simulink model "PowerFlow_lab_exercise_2024"  (R2024a)
settings: Solver=ode23tb  StartTime=0.0  StopTime=0.5  MaxStep=0.04  RelTol=1e-3  EnableMultiTasking=on
undefined symbols (not defined in the file): D1, Delta
libraries: spsThreePhaseVIMeasurementLib x11, spsLoadFlowBusLib x6, spsThreePhasePISectionLineLib x5, spsRMSLib x5, spsThreePhaseParallelRLCLoadLib x4, spsThreePhaseSourceLib x2, spsThreePhaseTransformerTwoWindingsLib x1, spspowerguiLib x1
Description:
  | Copyright 2008-2019 The MathWorks, Inc.
settings Model: Creator=MathWorks  LastModifiedBy=adysk
settings SolverCC: AlgebraicLoopSolver=TrustRegion
settings DataIOCC: LimitDataPoints=on  SaveFormat=Array  SignalLoggingSaveFormat=ModelDataLogs  ReturnWorkspaceOutputs=off
settings OptimizationCC: ExpressionDepthLimit=2147483647  LifeSpan=inf
settings DebuggingCC: UnderspecifiedInitializationDetection=Classic  MergeDetectMultiDrivingBlocksExec=none  SolverPrmCheckMsg=warning  FcnCallInpInsideContextMsg=warning  StateNameClashWarn=warning  SFUnexpectedBacktrackingDiag=warning  SFNoUnconditionalDefaultTransitionDiag=warning  SFExecutionAtInitializationDiag=none  ArithmeticOperatorsInVariantConditions=warning
settings HardwareCC: ProdBitPerPointer=32  ProdBitPerSizeT=32  ProdBitPerPtrDiffT=32  ProdLargestAtomicFloat=None  ProdIntDivRoundTo=Undefined  ProdEndianess=Unspecified  ProdWordSize=32  ProdHWDeviceType=32-bit Generic
settings ModelReferenceCC: EnableRefExpFcnMdlSchedulingChecks=on  PropagateSignalLabelsOutOfModel=off
settings SFSimCC: SimUseLocalCustomCode=off  CustomCodeUndefinedFunction=UseInterfaceOnly
settings RTWCC: RTWUseLocalCustomCode=off  GPUComputeCapability=3.5  DLArmComputeVersion=19.05
settings CodeAppCC: StateflowObjectComments=on
settings GRTTargetCC: TargetLangStandard=C89/C90 (ANSI)  CombineOutputUpdateFcns=off  GRTInterface=on
settings ConfigComp: CovMetricSettings=dw  CovSaveCumulativeToWorkspaceVar=on  CovSaveSingleToWorkspaceVar=on  CovExternalEMLEnable=off  CovSFcnEnable=off
settings SimscapeCC: SimscapeNormalizeSystem=off

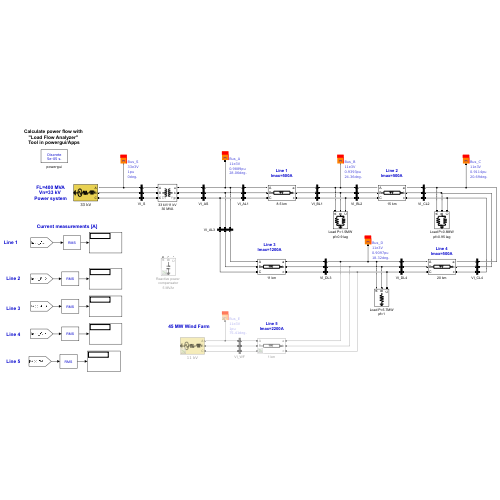
[thumbnail: Simulink's stored preview of the top-level diagram]
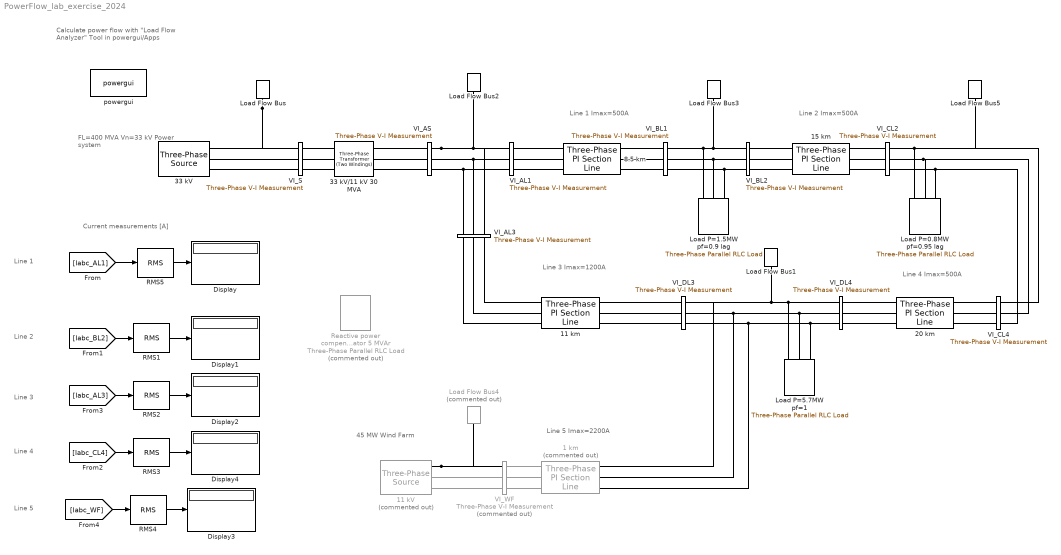
== system PowerFlow_lab_exercise_2024 ==
  note: Line 1
      | Imax=500A
  note: Current measurements [A]
  note: FL=400 MVA
      | Vn=33 kV
      | Power system
  note: Calculate power flow with
      | "Load Flow Analyzer"
      | Tool in powergui/Apps
  note: Line 2
      | Imax=500A
  note: Line 4
      | Imax=500A
  note: Line 3
      | Imax=1200A
  note: Line 1
  note: Line 2
  note: Line 3
  note: Line 4
  note: Line 5
  note: Line 5
      | Imax=2200A
  note: 45 MW Wind Farm
  1 km : spsThreePhasePISectionLineLib/Three-Phase PI Section Line  Commented=on  LConnTagsString=a|b|c  RConnTagsString=A|B|C  Length=1  Frequency=50  Resistances=[0.1153 0.413]  Inductances=[1.05e-3 3.32e-3]  Capacitances=[11.33e-009 5.01e-009]
  11 kV : spsThreePhaseSourceLib/Three-Phase Source  Commented=on  InternalConnection=Yg  VoltagePhases=off  Voltage=(11000)*1.29795  PhaseAngle=102.4466  Voltage_phases=[25e3 25e3 25e3]/sqrt(3)  PhaseAngles_phases=[0 -120 +120]  Frequency=50  NonIdealSource=on  SpecifyImpedance=on  Resistance=0.8929  Inductance=16.58e-3  ShortCircuitLevel=50e6  BaseVoltage=11e3  XRratio=7  BusType=PV  Pref=30000000  Qref=3000000  Prefabc=[10e3, 10e3, 10e3]  Qrefabc=[0, 0, 0]  Qmin=-20000000  Qmax=20000000
  11 km : spsThreePhasePISectionLineLib/Three-Phase PI Section Line  LConnTagsString=a|b|c  RConnTagsString=A|B|C  Length=11  Frequency=50  Resistances=[0.1153 0.413]  Inductances=[1.05e-3 3.32e-3]  Capacitances=[11.33e-009 5.01e-009]
  15 km : spsThreePhasePISectionLineLib/Three-Phase PI Section Line  LConnTagsString=a|b|c  RConnTagsString=A|B|C  Length=15  Frequency=50  Resistances=[0.1153 0.413]  Inductances=[1.05e-3 3.32e-3]  Capacitances=[11.33e-009 5.01e-009]
  20 km : spsThreePhasePISectionLineLib/Three-Phase PI Section Line  LConnTagsString=a|b|c  RConnTagsString=A|B|C  Length=20  Frequency=50  Resistances=[0.1153 0.413]  Inductances=[1.05e-3 3.32e-3]  Capacitances=[11.33e-009 5.01e-009]
  33 kV : spsThreePhaseSourceLib/Three-Phase Source  InternalConnection=Yg  VoltagePhases=off  Voltage=(33000)*1.00988  PhaseAngle=1.1485  Voltage_phases=[25e3 25e3 25e3]/sqrt(3)  PhaseAngles_phases=[0 -120 +120]  Frequency=50  NonIdealSource=on  SpecifyImpedance=on  Resistance=0.8929  Inductance=16.58e-3  ShortCircuitLevel=400e6  BaseVoltage=33e3  XRratio=7  BusType=swing  Pref=10000000  Qref=3000000  Prefabc=[10e3, 10e3, 10e3]  Qrefabc=[0, 0, 0]  Qmin=-Inf  Qmax=Inf
  33 kV/11 kV 30 MVA : spsThreePhaseTransformerTwoWindingsLib/Three-Phase Transformer (Two Windings)  Winding1Connection=Delta (D1)  Winding2Connection=Yg  CoreType=Three single-phase transformers  SetSaturation=off  Hysteresis=off  DataFile='basic_model'  SetInitialFlux=off  Measurements=None  UNITS=pu  NominalPower=[30e6 50 ]  Winding1="[33e3  0.002    0.06 ]"  Winding2="[ 11e3  0.002  0.06]"  Rm=5000  Lm=500  L0=0.5  Saturation="[ 0,0  ;  0.005,1.2  ;  1.0,1.4 ]"  InitialFluxes=[ 0.8 , -0.8 , 0.7 ]  BreakLoop=off  DiscreteSolver=Trapezoidal iterative  DataType=off  TransfoNumber=0
  8.5 km : spsThreePhasePISectionLineLib/Three-Phase PI Section Line  LConnTagsString=a|b|c  RConnTagsString=A|B|C  Length=8.5  Frequency=50  Resistances=[0.1153 0.413]  Inductances=[1.05e-3 3.32e-3]  Capacitances=[11.33e-009 5.01e-009]
  Display{,1..4} (5 alike) : Display
  Load Flow Bus : spsLoadFlowBusLib/Load Flow Bus  LConnTagsString=a  Phases=single  Connectors=on one side  ID=Bus_S  Vbase=33e3  Vref=1  Vangle=0  VLF=1  VLFb=1  VLFc=1  angleLF=0  angleLFb=0  angleLFc=0
      settings: AttributesFormatString=%<ID>\n%<Vbase>V\n%<VLF>pu\n%<angleLF>deg.
  Load Flow Bus1 : spsLoadFlowBusLib/Load Flow Bus  LConnTagsString=a  Phases=single  Connectors=on one side  ID=Bus_D  Vbase=11e3  Vref=1  Vangle=0  VLF=0.9097  VLFb=1  VLFc=1  angleLF=18.32  angleLFb=0  angleLFc=0
      settings: AttributesFormatString=%<ID>\n%<Vbase>V\n%<VLF>pu\n%<angleLF>deg.
  Load Flow Bus2 : spsLoadFlowBusLib/Load Flow Bus  LConnTagsString=a  Phases=single  Connectors=on one side  ID=Bus_A  Vbase=11e3  Vref=1  Vangle=0  VLF=0.9889  VLFb=1  VLFc=1  angleLF=28.06  angleLFb=0  angleLFc=0
      settings: AttributesFormatString=%<ID>\n%<Vbase>V\n%<VLF>pu\n%<angleLF>deg.
  Load Flow Bus3 : spsLoadFlowBusLib/Load Flow Bus  LConnTagsString=a  Phases=single  Connectors=on one side  ID=Bus_B  Vbase=11e3  Vref=1  Vangle=0  VLF=0.9393  VLFb=1  VLFc=1  angleLF=24.36  angleLFb=0  angleLFc=0
      settings: AttributesFormatString=%<ID>\n%<Vbase>V\n%<VLF>pu\n%<angleLF>deg.
  Load Flow Bus4 : spsLoadFlowBusLib/Load Flow Bus  Commented=on  LConnTagsString=a  Phases=single  Connectors=on one side  ID=Bus_E  Vbase=11e3  Vref=1.  Vangle=0  VLF=1  VLFb=1  VLFc=1  angleLF=75.41  angleLFb=0  angleLFc=0
      settings: AttributesFormatString=%<ID>\n%<Vbase>V\n%<VLF>pu\n%<angleLF>deg.
  Load Flow Bus5 : spsLoadFlowBusLib/Load Flow Bus  LConnTagsString=a  Phases=single  Connectors=on one side  ID=Bus_C  Vbase=11e3  Vref=1  Vangle=0  VLF=0.9114  VLFb=1  VLFc=1  angleLF=20.69  angleLFb=0  angleLFc=0
      settings: AttributesFormatString=%<ID>\n%<Vbase>V\n%<VLF>pu\n%<angleLF>deg.
  Load P=0.8MW pf=0.95 lag : spsThreePhaseParallelRLCLoadLib/Three-Phase Parallel RLC Load  LConnTagsString=A|B|C  Configuration=Y (grounded)  NominalVoltage=(11000)*0.911414  Vabc=[1e3 1e3 1e3]  Vabcp=[1e3 1e3 1e3]  NominalFrequency=50  UnbalancedPower=off  ActivePower=800000  InductivePower=262950  CapacitivePower=0  Pabc=[10e3 9e3 11e3]  QLabc=[100 90 110]  QCabc=[100 90 110]  Pabcp=[10e3 9e3 11e3]  QLabcp=[100 90 110]  QCabcp=[100 90 110]  Measurements=None  LoadType=constant PQ
  Load P=1.5MW pf=0.9 lag : spsThreePhaseParallelRLCLoadLib/Three-Phase Parallel RLC Load  LConnTagsString=A|B|C  Configuration=Y (grounded)  NominalVoltage=(11000)*0.939268  Vabc=[1e3 1e3 1e3]  Vabcp=[1e3 1e3 1e3]  NominalFrequency=50  UnbalancedPower=off  ActivePower=1500000  InductivePower=726500  CapacitivePower=0  Pabc=[10e3 9e3 11e3]  QLabc=[100 90 110]  QCabc=[100 90 110]  Pabcp=[10e3 9e3 11e3]  QLabcp=[100 90 110]  QCabcp=[100 90 110]  Measurements=None  LoadType=constant PQ
  Load P=5.7MW pf=1 : spsThreePhaseParallelRLCLoadLib/Three-Phase Parallel RLC Load  LConnTagsString=A|B|C  Configuration=Y (grounded)  NominalVoltage=(11000)*0.9097  Vabc=[1e3 1e3 1e3]  Vabcp=[1e3 1e3 1e3]  NominalFrequency=50  UnbalancedPower=off  ActivePower=5700000  InductivePower=0  CapacitivePower=0  Pabc=[10e3 9e3 11e3]  QLabc=[100 90 110]  QCabc=[100 90 110]  Pabcp=[10e3 9e3 11e3]  QLabcp=[100 90 110]  QCabcp=[100 90 110]  Measurements=None  LoadType=constant PQ
  RMS{1..5} (5 alike) : spsRMSLib/RMS  TrueRMS=on  Freq=50  RMSInit=120  Ts=0
  Reactive power compensator 5 MVAr : spsThreePhaseParallelRLCLoadLib/Three-Phase Parallel RLC Load  Commented=on  LConnTagsString=A|B|C  Configuration=Y (grounded)  NominalVoltage=(11000)*0.943215  Vabc=[1e3 1e3 1e3]  Vabcp=[1e3 1e3 1e3]  NominalFrequency=50  UnbalancedPower=off  ActivePower=0  InductivePower=0  CapacitivePower=5000000  Pabc=[10e3 9e3 11e3]  QLabc=[100 90 110]  QCabc=[100 90 110]  Pabcp=[10e3 9e3 11e3]  QLabcp=[100 90 110]  QCabcp=[100 90 110]  Measurements=None  LoadType=constant PQ
  VI_AL1 : spsThreePhaseVIMeasurementLib/Three-Phase V-I Measurement  VoltageMeasurement=phase-to-ground  SetLabelV=on  LabelV=Vabc_AL1  Vpu=off  VpuLL=off  CurrentMeasurement=yes  SetLabelI=on  LabelI=Iabc_AL1  Ipu=off  Pbase=10e6  Vbase=25e3  OutputType=Complex  PhasorSimulation=off  PSBequivalent=0
  VI_AL3 : spsThreePhaseVIMeasurementLib/Three-Phase V-I Measurement  VoltageMeasurement=phase-to-ground  SetLabelV=on  LabelV=Vabc_AL3  Vpu=off  VpuLL=off  CurrentMeasurement=yes  SetLabelI=on  LabelI=Iabc_AL3  Ipu=off  Pbase=10e6  Vbase=25e3  OutputType=Complex  PhasorSimulation=off  PSBequivalent=0
  VI_AS : spsThreePhaseVIMeasurementLib/Three-Phase V-I Measurement  VoltageMeasurement=phase-to-ground  SetLabelV=on  LabelV=Vabc_AS  Vpu=off  VpuLL=off  CurrentMeasurement=yes  SetLabelI=on  LabelI=Iabc_AS  Ipu=off  Pbase=10e6  Vbase=25e3  OutputType=Complex  PhasorSimulation=off  PSBequivalent=0
  VI_BL1 : spsThreePhaseVIMeasurementLib/Three-Phase V-I Measurement  VoltageMeasurement=phase-to-ground  SetLabelV=on  LabelV=Vabc_BL1  Vpu=off  VpuLL=off  CurrentMeasurement=yes  SetLabelI=on  LabelI=Iabc_BL1  Ipu=off  Pbase=10e6  Vbase=25e3  OutputType=Complex  PhasorSimulation=off  PSBequivalent=0
  VI_BL2 : spsThreePhaseVIMeasurementLib/Three-Phase V-I Measurement  VoltageMeasurement=phase-to-ground  SetLabelV=on  LabelV=Vabc_BL2  Vpu=off  VpuLL=off  CurrentMeasurement=yes  SetLabelI=on  LabelI=Iabc_BL2  Ipu=off  Pbase=10e6  Vbase=25e3  OutputType=Complex  PhasorSimulation=off  PSBequivalent=0
  VI_CL2 : spsThreePhaseVIMeasurementLib/Three-Phase V-I Measurement  VoltageMeasurement=phase-to-ground  SetLabelV=on  LabelV=Vabc_CL2  Vpu=off  VpuLL=off  CurrentMeasurement=yes  SetLabelI=on  LabelI=Iabc_CL2  Ipu=off  Pbase=10e6  Vbase=25e3  OutputType=Complex  PhasorSimulation=off  PSBequivalent=0
  VI_CL4 : spsThreePhaseVIMeasurementLib/Three-Phase V-I Measurement  VoltageMeasurement=phase-to-ground  SetLabelV=on  LabelV=Vabc_CL4  Vpu=off  VpuLL=off  CurrentMeasurement=yes  SetLabelI=on  LabelI=Iabc_CL4  Ipu=off  Pbase=10e6  Vbase=25e3  OutputType=Complex  PhasorSimulation=off  PSBequivalent=0
  VI_DL3 : spsThreePhaseVIMeasurementLib/Three-Phase V-I Measurement  VoltageMeasurement=phase-to-ground  SetLabelV=on  LabelV=Vabc_DL3  Vpu=off  VpuLL=off  CurrentMeasurement=yes  SetLabelI=on  LabelI=Iabc_DL3  Ipu=off  Pbase=10e6  Vbase=25e3  OutputType=Complex  PhasorSimulation=off  PSBequivalent=0
  VI_DL4 : spsThreePhaseVIMeasurementLib/Three-Phase V-I Measurement  VoltageMeasurement=phase-to-ground  SetLabelV=on  LabelV=Vabc_DL4  Vpu=off  VpuLL=off  CurrentMeasurement=yes  SetLabelI=on  LabelI=Iabc_DL4  Ipu=off  Pbase=10e6  Vbase=25e3  OutputType=Complex  PhasorSimulation=off  PSBequivalent=0
  VI_S : spsThreePhaseVIMeasurementLib/Three-Phase V-I Measurement  VoltageMeasurement=phase-to-ground  SetLabelV=on  LabelV=Vabc_S  Vpu=off  VpuLL=off  CurrentMeasurement=yes  SetLabelI=on  LabelI=Iabc_S  Ipu=off  Pbase=100e6  Vbase=120e3  OutputType=Complex  PhasorSimulation=off  PSBequivalent=0
  VI_WF : spsThreePhaseVIMeasurementLib/Three-Phase V-I Measurement  Commented=on  VoltageMeasurement=phase-to-ground  SetLabelV=on  LabelV=Vabc_WF  Vpu=off  VpuLL=off  CurrentMeasurement=yes  SetLabelI=on  LabelI=Iabc_WF  Ipu=off  Pbase=10e6  Vbase=25e3  OutputType=Complex  PhasorSimulation=off  PSBequivalent=0
  powergui : spspowerguiLib/powergui  Priority=1  SimulationMode=Discrete  SampleTime=50e-6  frequency=50  Iterations=50  frequencyindice=50  Pbase=100e6  ErrMax=0.0001  UnitsV=kV  UnitsW=MW  buscounter=0  FunctionMessages=off  echomessages=off  EnableUseOfTLC=off  CurrentSourceSwitches=off  DisableSnubberDevices=off  DisableRonSwitches=off  DisableVfSwitches=off  DisplayEquations=off  AutomaticDiscreteSolvers=off  SolverType=Tustin  Interpol=off  ExternalGateDelay=off  methode=off  Ts=100  x0status=blocks  SPID=off  SwTol=0  HookPort=off  NonlinearTolerance=0  nMaxIteration=15  ContinueOnMaxIteration=off  RestoreLinks=warning  ResistiveCurrentMeasurement=off  Frange=[0:2:500]  Ylog=off  Xlog=on  ShowGrid=off  save=off  variable=ZData  structure=0  ZoomFFT=off  StartTime=0.0  cycles=1  DisplayStyle=1  fundamental=60  FreqAxis=off  MaxFrequency=1000  frequencyindicesteady=1  RmsSteady=1  display=off
  wires:
  [Iabc_AL1] -> RMS5/1
  RMS5/1 -> Display/1
  RMS1/1 -> Display1/1
  [Iabc_BL2] -> RMS1/1
  RMS2/1 -> Display2/1
  RMS3/1 -> Display4/1
  [Iabc_AL3] -> RMS2/1
  [Iabc_CL4] -> RMS3/1
  [Iabc_WF] -> RMS4/1
  RMS4/1 -> Display3/1
  connections:
  VI_S/LConn3 -- 33 kV/RConn3
  VI_AS/LConn3 -- 33 kV/11 kV 30 MVA/RConn3
  VI_S/RConn1 -- 33 kV/11 kV 30 MVA/LConn1
  VI_BL1/RConn1 -- 8.5 km/RConn1
  VI_S/RConn3 -- 33 kV/11 kV 30 MVA/LConn3
  VI_S/RConn2 -- 33 kV/11 kV 30 MVA/LConn2
  Load Flow Bus/LConn1 -- VI_S/LConn1 -- 33 kV/RConn1
  VI_S/LConn2 -- 33 kV/RConn2
  VI_AS/LConn2 -- 33 kV/11 kV 30 MVA/RConn2
  VI_AS/RConn1 -- VI_AL3/LConn1 -- VI_AL1/LConn1 -- Load Flow Bus2/LConn1
  VI_CL2/RConn1 -- 15 km/RConn1
  VI_DL4/LConn1 -- Load P=5.7MW pf=1/LConn1 -- 1 km/RConn1 -- VI_DL3/LConn1 -- Load Flow Bus1/LConn1
  VI_DL3/LConn2 -- 1 km/RConn2 -- Load P=5.7MW pf=1/LConn2 -- VI_DL4/LConn2
  VI_DL3/LConn3 -- 1 km/RConn3 -- Load P=5.7MW pf=1/LConn3 -- VI_DL4/LConn3
  Load P=0.8MW pf=0.95 lag/LConn1 -- VI_CL4/LConn1 -- Load Flow Bus5/LConn1 -- VI_CL2/LConn1
  VI_CL2/LConn2 -- VI_CL4/LConn2 -- Load P=0.8MW pf=0.95 lag/LConn2
  Load P=0.8MW pf=0.95 lag/LConn3 -- VI_CL4/LConn3 -- VI_CL2/LConn3
  VI_AS/LConn1 -- 33 kV/11 kV 30 MVA/RConn1
  VI_AL3/RConn3 -- 11 km/LConn3
  VI_AL3/RConn2 -- 11 km/LConn2
  VI_AL3/RConn1 -- 11 km/LConn1
  VI_BL1/RConn2 -- 8.5 km/RConn2
  VI_BL1/RConn3 -- 8.5 km/RConn3
  VI_BL1/LConn3 -- Load P=1.5MW pf=0.9 lag/LConn3 -- VI_BL2/LConn3
  VI_BL1/LConn2 -- VI_BL2/LConn2 -- Load P=1.5MW pf=0.9 lag/LConn2
  VI_BL1/LConn1 -- Load P=1.5MW pf=0.9 lag/LConn1 -- Load Flow Bus3/LConn1 -- VI_BL2/LConn1
  VI_BL2/RConn1 -- 15 km/LConn1
  VI_BL2/RConn2 -- 15 km/LConn2
  VI_BL2/RConn3 -- 15 km/LConn3
  VI_CL2/RConn2 -- 15 km/RConn2
  VI_CL2/RConn3 -- 15 km/RConn3
  VI_DL4/RConn1 -- 20 km/LConn1
  VI_DL4/RConn2 -- 20 km/LConn2
  VI_DL4/RConn3 -- 20 km/LConn3
  VI_DL3/RConn1 -- 11 km/RConn1
  VI_DL3/RConn2 -- 11 km/RConn2
  VI_DL3/RConn3 -- 11 km/RConn3
  VI_AL1/RConn1 -- 8.5 km/LConn1
  VI_AL1/RConn2 -- 8.5 km/LConn2
  VI_AL1/RConn3 -- 8.5 km/LConn3
  VI_AL1/LConn2 -- VI_AL3/LConn2 -- VI_AS/RConn2
  VI_AL1/LConn3 -- VI_AL3/LConn3 -- VI_AS/RConn3
  11 kV/RConn1 -- Load Flow Bus4/LConn1 -- VI_WF/LConn1
  VI_WF/RConn2 -- 1 km/LConn2
  11 kV/RConn2 -- VI_WF/LConn2
  VI_WF/RConn3 -- 1 km/LConn3
  11 kV/RConn3 -- VI_WF/LConn3
  VI_WF/RConn1 -- 1 km/LConn1
  VI_CL4/RConn1 -- 20 km/RConn1
  VI_CL4/RConn2 -- 20 km/RConn2
  VI_CL4/RConn3 -- 20 km/RConn3
